simulink model "LQR"  (R2022a)
settings: Solver=VariableStepAuto  StartTime=0.0  StopTime=10.0  RelTol=1e-3
values from neighbouring files (symbols this model uses):
  dragConstants = [dx, dy, 0]    [parameters_init.m]    (also in parameters_init2.m)
  g = 9.81    [LQRCalcs.m]    (also in cf_firstOrderStateMdl.m; init_parameters.m; main.m; parameters_buildingSimulink.m)
  Gamma = [cT, cT, cT, cT ... (first row only)    [init_parameters.m]    (also in parameters_buildingSimulink.m; parameters_init.m; parameters_init2.m; parameters_init____CodeToImplementLater.m)
  GammaInv = inv(Gamma)    [init_parameters.m]    (also in parameters_buildingSimulink.m; parameters_init.m; parameters_init2.m)
  J = cat(2, [0 0 0]', J)    [LQRCalcs.m]    (also in init_parameters.m = diag([0.082, 0.0845, 0.1377]); main.m = diag([0.082, 0.0845, 0.1377]); parameters_buildingSimulink.m = diag([0.082, 0.0845, 0.1377]); parameters_init.m = Crazyflie.J)
  J_inv = inv(J)    [main.m]    (also in parameters_init.m; parameters_init2.m)
  m = 0.003    [LQRCalcs.m]    (also in cf_firstOrderStateMdl.m; init_parameters.m = 4.34; main.m = 4.34; parameters_buildingSimulink.m = 4.34)
  projectionMatrix = [1, 0, 0; 0, 1, 0]    [parameters_init.m]    (also in parameters_init2.m)
undefined symbols (not defined in the file or in its folder): Gain, sigbuilder_block
libraries: matrix_library x2, aerolibutil x2, sharedtransform x2
settings Model: Creator=Drew Lab Computer 1  LastModifiedBy=Drew Lab Computer 1

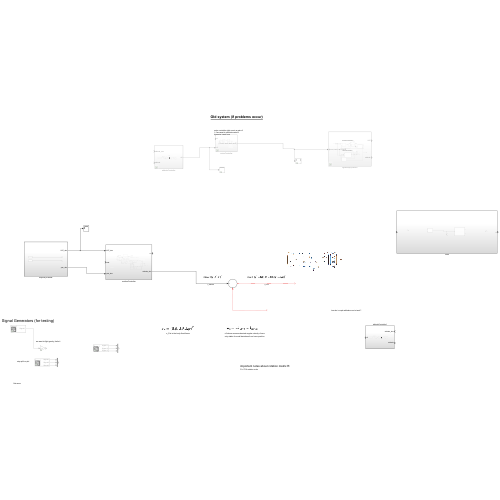
[thumbnail: Simulink's stored preview of the top-level diagram]
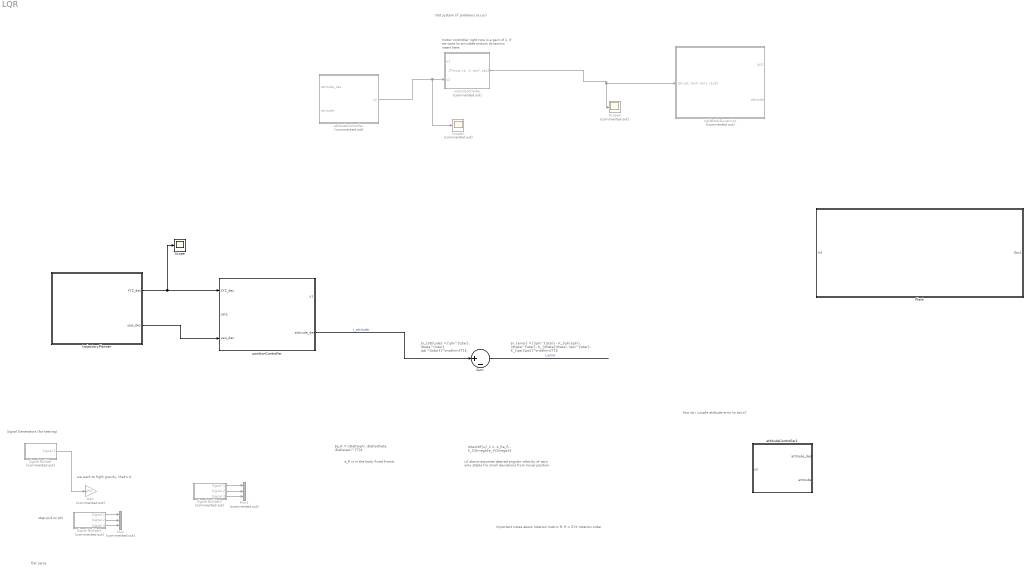
== system LQR ==
  note: $r_{attitude} = [\phi^{\star}, \theta^{\star}, \psi^{\star}]^\mathrm{T}$
  note: Old system (if problems occur)
  note: we want to fight gravity, that's it
  note: Signal Generators (for testing)
  note: flat zeros
  note: step pi/4 on phi
  note: $\textbf{u}_2 = -k_Re_R - k_{\Omega}e_{\Omega}$
  note: motor controller right now is a gain of 1, if we want to simulate motors dynamics insert here
  note: $e_R = (\Delta\phi, \Delta\theta, \Delta\psi)^{T}$
  note: $r_{error} = [(\phi^{\star} - K_{\phi}\phi), (\theta^{\star}- K_{\theta}\theta), (\psi^{\star}- K_{\psi}\psi)]^\mathrm{T}$
  note: u2 above assumes desired angular velocity of zero
      | only stable fro small deviations from hover position
  note: how do i couple attitude error to tau's?
  note: important notes about rotation matrix R:
      | R = ZYX rotation order
  note: e_R is in the body-fixed frame
  Gain : Gain  Commented=on  Gain=g*m
  Mux : Mux  Commented=on  Inputs=3
  Mux1 : Mux  Commented=on  Inputs=3
  Plant : Subsystem
  Scope : Scope
  Scope2 : Scope  Commented=on
  Scope3 : Scope  Commented=on
  Signal Builder : Subsystem  Tag=STV Subsys  Commented=on  LoadFcn=sigbuilder_block('load');  StartFcn=sigbuilder_block('start');  StopFcn=sigbuilder_block('stop');  ClipboardFcn=sigbuilder_block('clipboard');  mask(Sigbuilder block){tuvar=[0:10]}
      mask help: Simulink:masks:SigbuilderBlock_MD
      mask init:
      | if ~strcmp(get_param(bdroot(gcbh),'SimulationStatus'),'stopped') tuvar = sigbuilder_block('maskInit'); end
      settings: CopyFcn=sigbuilder_block('copy');  DeleteFcn=sigbuilder_block('delete');  ModelCloseFcn=sigbuilder_block('modelClose');  PreSaveFcn=sigbuilder_block('preSave');  PauseFcn=sigbuilder_block('pause');  ContinueFcn=sigbuilder_block('continue');  NameChangeFcn=sigbuilder_block('namechange');  OpenFcn=sigbuilder_block('open',[437.6 199.2 550.4 400 ]);  CloseFcn=sigbuilder_block('close');
      mask Display: plot(0, 0, 100, 100,[2, 2, 32, 32, 2], [68, 8, 8, 68, 68],[32, 2], [38, 38], [32, 19, 2],[53, 60, 44], [32, 17, 17, 2],[16, 16, 31, 31]);txt = getActiveGroup(gcbh);text(2, 100, txt,'verticalAlignment', 'top');
  Signal Builder1 : Subsystem  Tag=STV Subsys  Commented=on  LoadFcn=sigbuilder_block('load');  StartFcn=sigbuilder_block('start');  StopFcn=sigbuilder_block('stop');  ClipboardFcn=sigbuilder_block('clipboard');  mask(Sigbuilder block){tuvar=[0:10]}
      mask help: Simulink:masks:SigbuilderBlock_MD
      mask init:
      | if ~strcmp(get_param(bdroot(gcbh),'SimulationStatus'),'stopped') tuvar = sigbuilder_block('maskInit'); end
      settings: CopyFcn=sigbuilder_block('copy');  DeleteFcn=sigbuilder_block('delete');  ModelCloseFcn=sigbuilder_block('modelClose');  PreSaveFcn=sigbuilder_block('preSave');  PauseFcn=sigbuilder_block('pause');  ContinueFcn=sigbuilder_block('continue');  NameChangeFcn=sigbuilder_block('namechange');  OpenFcn=sigbuilder_block('open',[437.6 199.2 550.4 400 ]);  CloseFcn=sigbuilder_block('close');
      mask Display: plot(0, 0, 100, 100,[2, 2, 32, 32, 2], [68, 8, 8, 68, 68],[32, 2], [38, 38], [32, 19, 2],[53, 60, 44], [32, 17, 17, 2],[16, 16, 31, 31]);txt = getActiveGroup(gcbh);text(2, 100, txt,'verticalAlignment', 'top');
  Signal Builder2 : Subsystem  Tag=STV Subsys  Commented=on  LoadFcn=sigbuilder_block('load');  StartFcn=sigbuilder_block('start');  StopFcn=sigbuilder_block('stop');  ClipboardFcn=sigbuilder_block('clipboard');  mask(Sigbuilder block){tuvar=[0:10]}
      mask help: Simulink:masks:SigbuilderBlock_MD
      mask init:
      | if ~strcmp(get_param(bdroot(gcbh),'SimulationStatus'),'stopped') tuvar = sigbuilder_block('maskInit'); end
      settings: CopyFcn=sigbuilder_block('copy');  DeleteFcn=sigbuilder_block('delete');  ModelCloseFcn=sigbuilder_block('modelClose');  PreSaveFcn=sigbuilder_block('preSave');  PauseFcn=sigbuilder_block('pause');  ContinueFcn=sigbuilder_block('continue');  NameChangeFcn=sigbuilder_block('namechange');  OpenFcn=sigbuilder_block('open',[437.6 199.2 550.4 400 ]);  CloseFcn=sigbuilder_block('close');
      mask Display: plot(0, 0, 100, 100,[2, 2, 32, 32, 2], [68, 8, 8, 68, 68],[32, 2], [38, 38], [32, 19, 2],[53, 60, 44], [32, 17, 17, 2],[16, 16, 31, 31]);txt = getActiveGroup(gcbh);text(2, 100, txt,'verticalAlignment', 'top');
  Sum : Sum  Inputs=|+-
  attitudeController : Subsystem  Commented=on
  attitudeController1 : Subsystem
  motorController : Subsystem  Commented=on
  positionController : Subsystem
  rigidBodyDynamics : Subsystem  Commented=on
  trajectoryPlanner : Subsystem
  wires:
  Sum/1 -> ?  "r_error"
  Signal Builder/1(Signal 1) -> Gain/1
  Signal Builder2/1(Signal 1) -> Mux1/1
  Signal Builder2/3(Signal 3) -> Mux1/3
  Signal Builder2/2(Signal 2) -> Mux1/2
  trajectoryPlanner/1(XYZ_des) -> Scope/1, positionController/1(XYZ_des)
  Signal Builder1/1(Signal 1) -> Mux/1
  Signal Builder1/3(Signal 3) -> Mux/3
  positionController/2(attitude_des) -> Sum/1  "r_attitude"
  Signal Builder1/2(Signal 2) -> Mux/2
  motorController/1("[Thrust, tauX, tauY, tauZ]") -> Scope3/1, rigidBodyDynamics/1("[thrust, tauX, tauY, tauZ]")
  attitudeController/1(u2) -> Scope2/1, motorController/2(u2)
  trajectoryPlanner/2(yaw_des) -> positionController/3(yaw_des)
  ? -> Sum/2

== system LQR/Plant ==
  In1 : Inport
  Scope1 : Scope
  motorController1 : Subsystem
  rigidBodyDynamics1 : Subsystem
  Out1 : Outport
  wires:
  motorController1/1("[Thrust, tauX, tauY, tauZ]") -> Scope1/1, rigidBodyDynamics1/1("[thrust, tauX, tauY, tauZ]")

== system LQR/Signal Builder ==
  Demux : Demux  Tag=STV Demux  Outputs=1
      settings: DisplayOption=none
  FromWs : FromWorkspace  Tag=STV FromWs  VariableName=tuvar
      SigBuilderData=|
      | common.afterFinalStr = 'Extrapolate'
      | common.sampleTime = 0
      | dataSet.timeRange = [0 10]
      | dataSet.name = 'Group 1'
      | sbobj.Groups.Name = 'Group 1'
      | sbobj.Groups.Signals.Name = 'Signal 1'
      | sbobj.Groups.Signals.XData = [0 10]
      | sbobj.Groups.Signals.YData = [1 1]
  Signal 1 : Outport  Tag=STV Outport
  wires:
  Demux/1 -> Signal 1/1
  FromWs/1 -> Demux/1

== system LQR/Signal Builder1 ==
  Demux : Demux  Tag=STV Demux  Outputs=3
      settings: DisplayOption=none
  FromWs : FromWorkspace  Tag=STV FromWs  VariableName=tuvar
      SigBuilderData=|
      | common.afterFinalStr = 'Extrapolate'
      | common.sampleTime = 0
      | dataSet.timeRange = [0 10]
      | dataSet.name = 'Group 1'
      | sbobj.Groups.Name = 'Group 1'
      | sbobj.Groups.Signals(1).Name = 'Signal 1'
      | sbobj.Groups.Signals(1).XData = [0 1 1 10]
      | sbobj.Groups.Signals(1).YData = [0 0 0.1 0.1]
      | sbobj.Groups.Signals(2).Name = 'Signal 2'
      | sbobj.Groups.Signals(2).XData = [0 10]
      | sbobj.Groups.Signals(2).YData = [0 0]
      | sbobj.Groups.Signals(3).Name = 'Signal 3'
      | sbobj.Groups.Signals(3).XData = [0 10]
      | sbobj.Groups.Signals(3).YData = [0 0]
  Signal 1 : Outport  Tag=STV Outport
  Signal 2 : Outport  Tag=STV Outport  Port=2
  Signal 3 : Outport  Tag=STV Outport  Port=3
  wires:
  Demux/1 -> Signal 1/1
  FromWs/1 -> Demux/1
  Demux/2 -> Signal 2/1
  Demux/3 -> Signal 3/1

== system LQR/Signal Builder2 ==
  Demux : Demux  Tag=STV Demux  Outputs=3
      settings: DisplayOption=none
  FromWs : FromWorkspace  Tag=STV FromWs  VariableName=tuvar
      SigBuilderData=|
      | common.afterFinalStr = 'Extrapolate'
      | common.sampleTime = 0
      | dataSet.timeRange = [0 10]
      | dataSet.name = 'Group 1'
      | sbobj.Groups.Name = 'Group 1'
      | sbobj.Groups.Signals(1).Name = 'Signal 1'
      | sbobj.Groups.Signals(1).XData = [0 10]
      | sbobj.Groups.Signals(1).YData = [0 0]
      | sbobj.Groups.Signals(2).Name = 'Signal 2'
      | sbobj.Groups.Signals(2).XData = [0 10]
      | sbobj.Groups.Signals(2).YData = [0 0]
      | sbobj.Groups.Signals(3).Name = 'Signal 3'
      | sbobj.Groups.Signals(3).XData = [0 10]
      | sbobj.Groups.Signals(3).YData = [0 0]
  Signal 1 : Outport  Tag=STV Outport
  Signal 2 : Outport  Tag=STV Outport  Port=2
  Signal 3 : Outport  Tag=STV Outport  Port=3
  wires:
  Demux/1 -> Signal 1/1
  FromWs/1 -> Demux/1
  Demux/2 -> Signal 2/1
  Demux/3 -> Signal 3/1

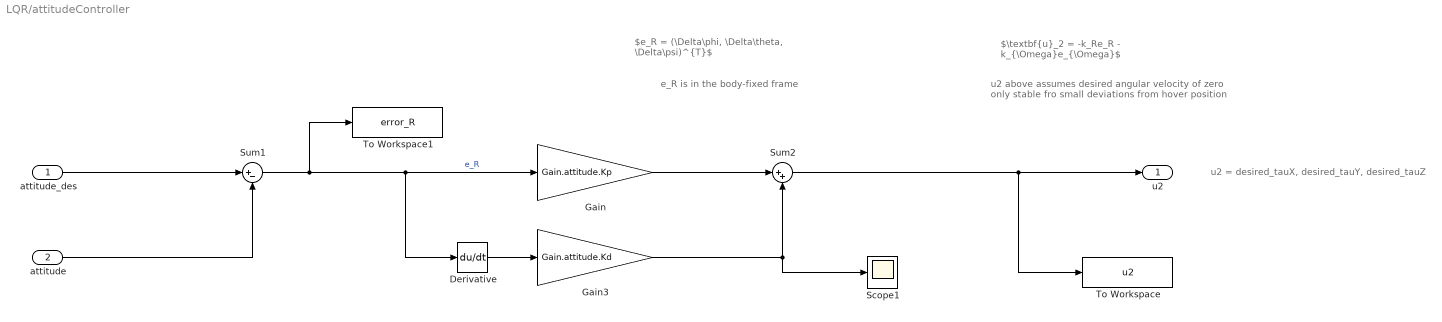
== system LQR/attitudeController ==
  note: u2 above assumes desired angular velocity of zero
      | only stable fro small deviations from hover position
  note: e_R is in the body-fixed frame
  note: $e_R = (\Delta\phi, \Delta\theta, \Delta\psi)^{T}$
  note: $\textbf{u}_2 = -k_Re_R - k_{\Omega}e_{\Omega}$
  note: u2 = desired_tauX, desired_tauY, desired_tauZ
  attitude_des : Inport
  attitude : Inport  Port=2
  Derivative : Derivative
  Gain : Gain  Gain=Gain.attitude.Kp
  Gain3 : Gain  Gain=Gain.attitude.Kd
  Scope1 : Scope
  Sum1 : Sum  Inputs=|+-
  Sum2 : Sum  Inputs=|++
  To Workspace : ToWorkspace  VariableName=u2  SaveFormat=Timeseries  SampleTime=-1
  To Workspace1 : ToWorkspace  VariableName=error_R  SaveFormat=Timeseries  SampleTime=-1
  u2 : Outport
  wires:
  attitude/1 -> Sum1/2
  Sum1/1 -> To Workspace1/1, Derivative/1, Gain/1  "e_R"
  Derivative/1 -> Gain3/1
  Gain/1 -> Sum2/1
  Gain3/1 -> Sum2/2, Scope1/1
  attitude_des/1 -> Sum1/1
  Sum2/1 -> To Workspace/1, u2/1

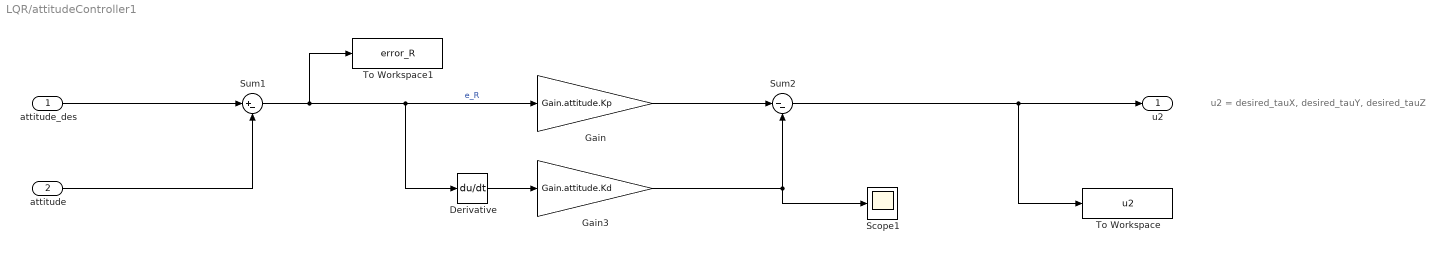
== system LQR/attitudeController1 ==
  note: u2 = desired_tauX, desired_tauY, desired_tauZ
  attitude_des : Inport
  attitude : Inport  Port=2
  Derivative : Derivative
  Gain : Gain  Gain=Gain.attitude.Kp
  Gain3 : Gain  Gain=Gain.attitude.Kd
  Scope1 : Scope
  Sum1 : Sum  Inputs=|+-
  Sum2 : Sum  Inputs=|--
  To Workspace : ToWorkspace  VariableName=u2  SaveFormat=Timeseries  SampleTime=-1
  To Workspace1 : ToWorkspace  VariableName=error_R  SaveFormat=Timeseries  SampleTime=-1
  u2 : Outport
  wires:
  attitude/1 -> Sum1/2
  Sum1/1 -> To Workspace1/1, Derivative/1, Gain/1  "e_R"
  Derivative/1 -> Gain3/1
  Gain/1 -> Sum2/1
  Gain3/1 -> Sum2/2, Scope1/1
  attitude_des/1 -> Sum1/1
  Sum2/1 -> To Workspace/1, u2/1

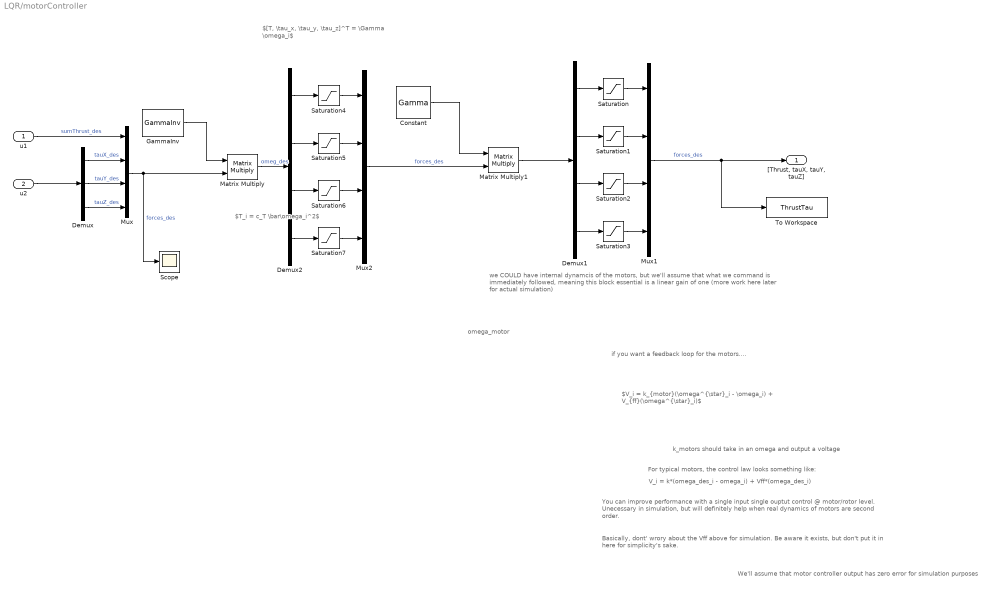
== system LQR/motorController ==
  note: $[T, \tau_x, \tau_y, \tau_z]^T = \Gamma \omega_i$
  note: if you want a feedback loop for the motors....
  note: we COULD have internal dynamcis of the motors, but we'll assume that what we command is immediately followed, meaning this block essential is a linear gain of one
      |
      | (more work here later for actual simulation)
  note: $T_i = c_T \bar\omega_i^2$
  note: omega_motor
  note: We'll assume that motor controller output has zero error for simulation purposes
  note: k_motors should take in an omega and output a voltage
  note: Basically, dont' wrory about the Vff above for simulation. Be aware it exists, but don't put it in here for simplicity's sake.
  note: You can improve performance with a single input single ouptut control @ motor/rotor level. Unecessary in simulation, but will definitely help when real dynamics of motors are second order.
  note: V_i = k*(omega_des_i - omega_i) + Vff*(omega_des_i)
  note: For typical motors, the control law looks something like:
  note: $V_i = k_{motor}(\omega^{\star}_i - \omega_i) + V_{ff}(\omega^{\star}_i)$
  u1 : Inport
  u2 : Inport  Port=2
  Constant : Constant  Value=Gamma
  Demux : Demux  Outputs=3
  Demux1 : Demux
  Demux2 : Demux
  GammaInv : Constant  Value=GammaInv
  Matrix Multiply : Product  Multiplication=Matrix(*)
  Matrix Multiply1 : Product  Multiplication=Matrix(*)
  Mux : Mux
  Mux1 : Mux
  Mux2 : Mux
  Saturation : Saturate  UpperLimit=Gain.saturation.attitude.Thrust(1)  LowerLimit=Gain.saturation.attitude.Thrust(2)
  Saturation1 : Saturate  UpperLimit=Gain.saturation.attitude.tauX(1)  LowerLimit=Gain.saturation.attitude.tauX(2)
  Saturation2 : Saturate  UpperLimit=Gain.saturation.attitude.tauY(1)  LowerLimit=Gain.saturation.attitude.tauY(2)  LinearizeAsGain=off
  Saturation3 : Saturate  UpperLimit=Gain.saturation.attitude.tauZ(1)  LowerLimit=Gain.saturation.attitude.tauZ(2)
  Saturation4 : Saturate  UpperLimit=Gain.saturation.attitude.Thrust(1)  LowerLimit=Gain.saturation.attitude.Thrust(2)
  Saturation5 : Saturate  UpperLimit=Gain.saturation.attitude.tauX(1)  LowerLimit=Gain.saturation.attitude.tauX(2)
  Saturation6 : Saturate  UpperLimit=Gain.saturation.attitude.tauY(1)  LowerLimit=Gain.saturation.attitude.tauY(2)  LinearizeAsGain=off
  Saturation7 : Saturate  UpperLimit=Gain.saturation.attitude.tauZ(1)  LowerLimit=Gain.saturation.attitude.tauZ(2)
  Scope : Scope
  To Workspace : ToWorkspace  VariableName=ThrustTau  SaveFormat=Timeseries  SampleTime=-1
  "[Thrust, tauX, tauY, tauZ]" : Outport
  wires:
  u2/1 -> Demux/1
  u1/1 -> Mux/1  "sumThrust_des"
  Demux/2 -> Mux/3  "tauY_des"
  Demux/1 -> Mux/2  "tauX_des"
  Demux/3 -> Mux/4  "tauZ_des"
  Mux/1 -> Matrix Multiply/2, Scope/1  "forces_des"
  GammaInv/1 -> Matrix Multiply/1
  Matrix Multiply/1 -> Demux2/1  "omeg_des"
  Constant/1 -> Matrix Multiply1/1
  Mux1/1 -> To Workspace/1, "[Thrust, tauX, tauY, tauZ]"/1  "forces_des"
  Demux1/1 -> Saturation/1
  Saturation/1 -> Mux1/1
  Demux1/2 -> Saturation1/1
  Demux1/3 -> Saturation2/1
  Demux1/4 -> Saturation3/1
  Saturation1/1 -> Mux1/2
  Saturation2/1 -> Mux1/3
  Saturation3/1 -> Mux1/4
  Matrix Multiply1/1 -> Demux1/1
  Demux2/2 -> Saturation5/1
  Demux2/4 -> Saturation7/1
  Saturation7/1 -> Mux2/4
  Demux2/1 -> Saturation4/1
  Demux2/3 -> Saturation6/1
  Saturation4/1 -> Mux2/1
  Saturation5/1 -> Mux2/2
  Saturation6/1 -> Mux2/3
  Mux2/1 -> Matrix Multiply1/2  "forces_des"

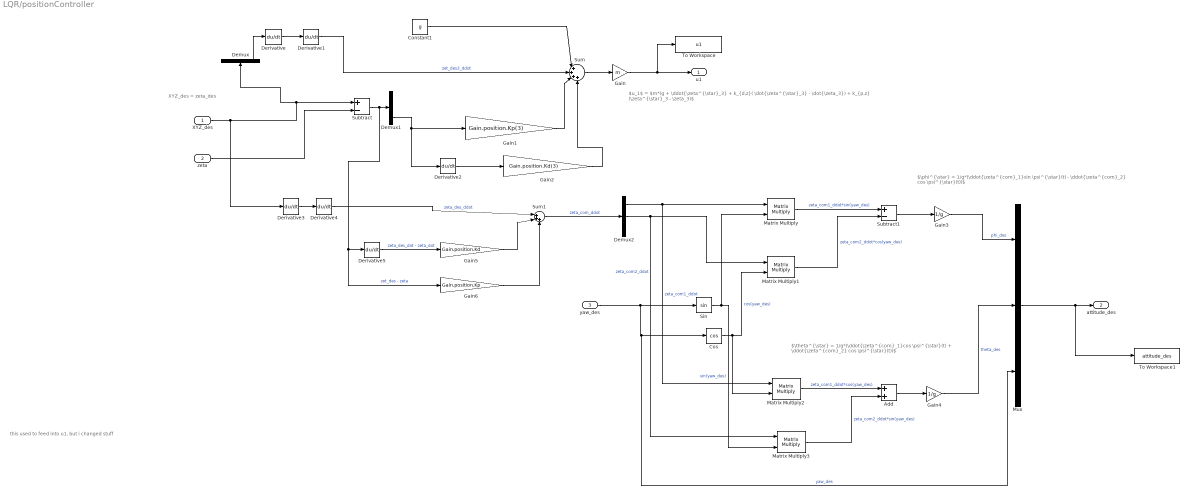
== system LQR/positionController ==
  note: $\theta^{\star} = 1/g*(\ddot{\zeta^{com}_1}cos \psi^{\star}(t) + \ddot{\zeta^{com}_2} cos \psi^{\star}(t))$
  note: $\phi^{\star} = 1/g*(\ddot{\zeta^{com}_1}sin \psi^{\star}(t) - \ddot{\zeta^{com}_2} cos \psi^{\star}(t))$
  note: XYZ_des = zeta_des
  note: $u_1$ = $m*(g + \ddot{\zeta^{\star}_3} + k_{d,z}( \dot{\zeta^{\star}_3} - \dot{\zeta_3}) + k_{p,z} (\zeta^{\star}_3 - \zeta_3)$
  note: this used to feed into u1, but i changed stuff
  XYZ_des : Inport
  zeta : Inport  Port=2
  yaw_des : Inport  Port=3
  Add : Sum
  Constant1 : Constant  Value=g
  Cos : Trigonometry  Operator=cos
  Demux : Demux  Outputs=3
  Demux1 : Demux  Outputs=3
  Demux2 : Demux  Outputs=3
  Derivative{,1..5} (6 alike) : Derivative
  Gain : Gain  Gain=m
  Gain1 : Gain  Gain=Gain.position.Kp(3)
  Gain2 : Gain  Gain=Gain.position.Kd(3)
  Gain3 : Gain  Gain=1/g
  Gain4 : Gain  Gain=1/g
  Gain5 : Gain  Gain=Gain.position.Kd
  Gain6 : Gain  Gain=Gain.position.Kp
  Matrix Multiply{,1..3} (4 alike) : Product  Multiplication=Matrix(*)
  Mux : Mux  Inputs=3
  Sin : Trigonometry
  Subtract : Sum  Inputs=+-
  Subtract1 : Sum  Inputs=+-
  Sum : Sum  Inputs=|++++
  Sum1 : Sum  Inputs=|+++
  To Workspace : ToWorkspace  VariableName=u1  SaveFormat=Timeseries  SampleTime=-1
  To Workspace1 : ToWorkspace  VariableName=attitude_des  SaveFormat=Timeseries  SampleTime=-1
  u1 : Outport
  attitude_des : Outport  Port=2
  wires:
  zeta/1 -> Subtract/2
  Sum/1 -> Gain/1
  Constant1/1 -> Sum/1
  XYZ_des/1 -> Derivative3/1, Subtract/1, Demux/1
  Demux/3 -> Derivative/1
  Derivative/1 -> Derivative1/1
  Derivative1/1 -> Sum/2  "zet_des3_ddot"
  Subtract/1 -> Gain6/1, Derivative5/1, Demux1/1  "zet_des - zeta"
  Demux1/3 -> Gain1/1, Derivative2/1
  Derivative2/1 -> Gain2/1
  Gain1/1 -> Sum/3
  Gain2/1 -> Sum/4
  Gain/1 -> To Workspace/1, u1/1
  Derivative3/1 -> Derivative4/1
  Derivative4/1 -> Sum1/1  "zeta_des_ddot"
  Derivative5/1 -> Gain5/1  "zeta_des_dot - zeta_dot"
  Gain5/1 -> Sum1/2
  Gain6/1 -> Sum1/3
  Sum1/1 -> Demux2/1  "zeta_com_ddot"
  yaw_des/1 -> Mux/3, Cos/1, Sin/1  "yaw_des"
  Demux2/1 -> Matrix Multiply2/1, Matrix Multiply/1  "zeta_com1_ddot"
  Sin/1 -> Matrix Multiply/2, Matrix Multiply3/2  "sin(yaw_des)"
  Matrix Multiply/1 -> Subtract1/1  "zeta_com1_ddot*sin(yaw_des)"
  Demux2/2 -> Matrix Multiply3/1, Matrix Multiply1/1  "zeta_com2_ddot"
  Cos/1 -> Matrix Multiply2/2, Matrix Multiply1/2  "cos(yaw_des)"
  Matrix Multiply1/1 -> Subtract1/2  "zeta_com2_ddot*cos(yaw_des)"
  Subtract1/1 -> Gain3/1
  Matrix Multiply2/1 -> Add/1  "zeta_com1_ddot*cos(yaw_des)"
  Matrix Multiply3/1 -> Add/2  "zeta_com2_ddot*sin(yaw_des)"
  Add/1 -> Gain4/1
  Gain3/1 -> Mux/1  "phi_des"
  Gain4/1 -> Mux/2  "theta_des"
  Mux/1 -> To Workspace1/1, attitude_des/1

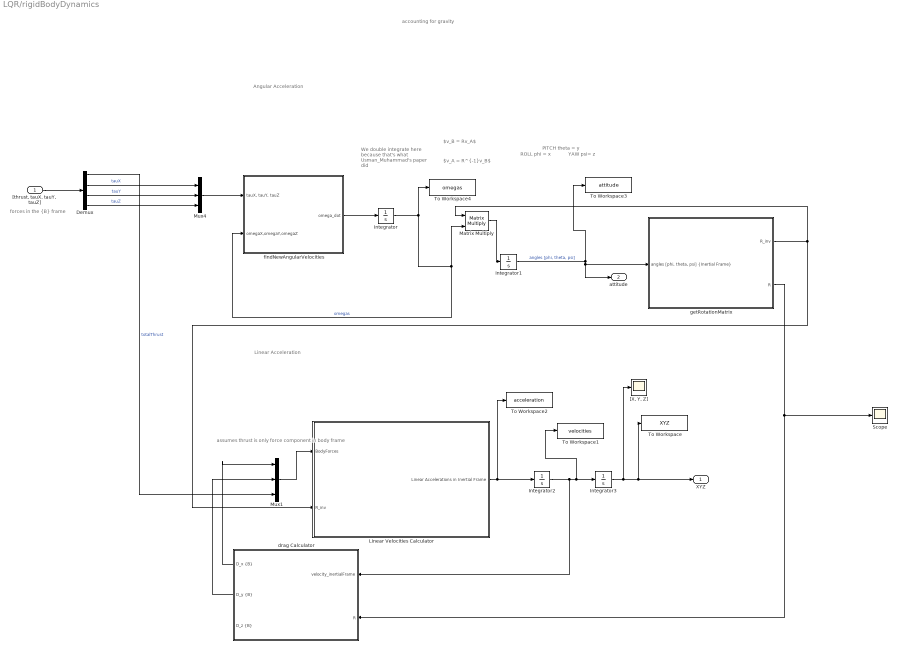
== system LQR/rigidBodyDynamics ==
  note: $v_A = R^{-1}v_B$
  note: assumes thrust is only force component in body frame
  note: We double integrate here because that's what Usman_Muhammad's paper did
  note: Angular Acceleration
  note: Linear Acceleration
  note: accounting for gravity
  note: forces in the {B} frame
  note: ROLL
      | phi = x
  note: PITCH
      | theta = y
  note: YAW
      | psi= z
  note: $v_B = Rv_A$
  "[thrust, tauX, tauY, tauZ]" : Inport
  Demux : Demux
  Integrator{,1..3} (4 alike) : Integrator
  Linear Velocities Calculator : Subsystem
  Matrix Multiply : Product  Multiplication=Matrix(*)
  Mux1 : Mux  Inputs=3
  Mux4 : Mux  Inputs=3
  Scope : Scope
  To Workspace : ToWorkspace  VariableName=XYZ  SaveFormat=Timeseries  SampleTime=-1
  To Workspace1 : ToWorkspace  VariableName=velocities  SaveFormat=Timeseries  SampleTime=-1
  To Workspace2 : ToWorkspace  VariableName=acceleration  SaveFormat=Timeseries  SampleTime=-1
  To Workspace3 : ToWorkspace  VariableName=attitude  SaveFormat=Timeseries  SampleTime=-1
  To Workspace4 : ToWorkspace  VariableName=omegas  SaveFormat=Timeseries  SampleTime=-1
  "[X, Y, Z]" : Scope
  drag Calculator : Subsystem
  findNewAngularVelocities : Subsystem
  getRotationMatrix : Subsystem
  XYZ : Outport
  attitude : Outport  Port=2
  wires:
  Demux/2 -> Mux4/1  "tauX"
  Demux/4 -> Mux4/3  "tauZ"
  Demux/3 -> Mux4/2  "tauY"
  "[thrust, tauX, tauY, tauZ]"/1 -> Demux/1
  Integrator1/1 -> attitude/1, getRotationMatrix/1("angles [phi, theta, psi] {Inertial Frame}"), To Workspace3/1  "angles [phi, theta, psi]"
  findNewAngularVelocities/1(omega_dot) -> Integrator/1
  Integrator/1 -> Matrix Multiply/2, findNewAngularVelocities/2(omegaX,omegaY,omegaZ), To Workspace4/1  "omegas"
  Mux4/1 -> findNewAngularVelocities/1("tauX, tauY, tauZ")
  Mux1/1 -> Linear Velocities Calculator/1(BodyForces)
  getRotationMatrix/1(R_inv) -> Linear Velocities Calculator/2(R_inv), Matrix Multiply/1
  Demux/1 -> Mux1/3  "totalThrust"
  Matrix Multiply/1 -> Integrator1/1
  Linear Velocities Calculator/1(Linear Accelerations in Inertial Frame) -> Integrator2/1, To Workspace2/1
  Integrator2/1 -> drag Calculator/1(velocity_inertialFrame), To Workspace1/1, Integrator3/1
  Integrator3/1 -> "[X, Y, Z]"/1, To Workspace/1, XYZ/1
  getRotationMatrix/2(R) -> Scope/1, drag Calculator/2(R)
  drag Calculator/1("D_x {B}") -> Mux1/1
  drag Calculator/2("D_y {B}") -> Mux1/2

== system LQR/trajectoryPlanner ==
  From Workspace : FromWorkspace  VariableName=zeta_des
  From Workspace1 : FromWorkspace  VariableName=yaw_des
  XYZ_des : Outport
  yaw_des : Outport  Port=2
  wires:
  From Workspace/1 -> XYZ_des/1
  From Workspace1/1 -> yaw_des/1

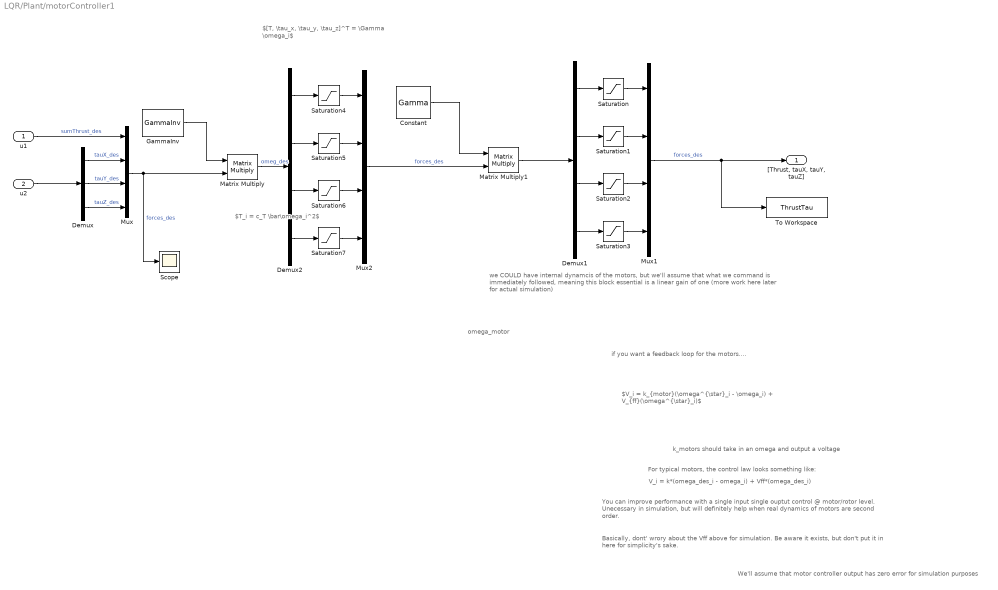
== system LQR/Plant/motorController1 ==
  note: $[T, \tau_x, \tau_y, \tau_z]^T = \Gamma \omega_i$
  note: if you want a feedback loop for the motors....
  note: we COULD have internal dynamcis of the motors, but we'll assume that what we command is immediately followed, meaning this block essential is a linear gain of one
      |
      | (more work here later for actual simulation)
  note: $T_i = c_T \bar\omega_i^2$
  note: omega_motor
  note: We'll assume that motor controller output has zero error for simulation purposes
  note: k_motors should take in an omega and output a voltage
  note: Basically, dont' wrory about the Vff above for simulation. Be aware it exists, but don't put it in here for simplicity's sake.
  note: You can improve performance with a single input single ouptut control @ motor/rotor level. Unecessary in simulation, but will definitely help when real dynamics of motors are second order.
  note: V_i = k*(omega_des_i - omega_i) + Vff*(omega_des_i)
  note: For typical motors, the control law looks something like:
  note: $V_i = k_{motor}(\omega^{\star}_i - \omega_i) + V_{ff}(\omega^{\star}_i)$
  u1 : Inport
  u2 : Inport  Port=2
  Constant : Constant  Value=Gamma
  Demux : Demux  Outputs=3
  Demux1 : Demux
  Demux2 : Demux
  GammaInv : Constant  Value=GammaInv
  Matrix Multiply : Product  Multiplication=Matrix(*)
  Matrix Multiply1 : Product  Multiplication=Matrix(*)
  Mux : Mux
  Mux1 : Mux
  Mux2 : Mux
  Saturation : Saturate  UpperLimit=Gain.saturation.attitude.Thrust(1)  LowerLimit=Gain.saturation.attitude.Thrust(2)
  Saturation1 : Saturate  UpperLimit=Gain.saturation.attitude.tauX(1)  LowerLimit=Gain.saturation.attitude.tauX(2)
  Saturation2 : Saturate  UpperLimit=Gain.saturation.attitude.tauY(1)  LowerLimit=Gain.saturation.attitude.tauY(2)  LinearizeAsGain=off
  Saturation3 : Saturate  UpperLimit=Gain.saturation.attitude.tauZ(1)  LowerLimit=Gain.saturation.attitude.tauZ(2)
  Saturation4 : Saturate  UpperLimit=Gain.saturation.attitude.Thrust(1)  LowerLimit=Gain.saturation.attitude.Thrust(2)
  Saturation5 : Saturate  UpperLimit=Gain.saturation.attitude.tauX(1)  LowerLimit=Gain.saturation.attitude.tauX(2)
  Saturation6 : Saturate  UpperLimit=Gain.saturation.attitude.tauY(1)  LowerLimit=Gain.saturation.attitude.tauY(2)  LinearizeAsGain=off
  Saturation7 : Saturate  UpperLimit=Gain.saturation.attitude.tauZ(1)  LowerLimit=Gain.saturation.attitude.tauZ(2)
  Scope : Scope
  To Workspace : ToWorkspace  VariableName=ThrustTau  SaveFormat=Timeseries  SampleTime=-1
  "[Thrust, tauX, tauY, tauZ]" : Outport
  wires:
  u2/1 -> Demux/1
  u1/1 -> Mux/1  "sumThrust_des"
  Demux/2 -> Mux/3  "tauY_des"
  Demux/1 -> Mux/2  "tauX_des"
  Demux/3 -> Mux/4  "tauZ_des"
  Mux/1 -> Matrix Multiply/2, Scope/1  "forces_des"
  GammaInv/1 -> Matrix Multiply/1
  Matrix Multiply/1 -> Demux2/1  "omeg_des"
  Constant/1 -> Matrix Multiply1/1
  Mux1/1 -> To Workspace/1, "[Thrust, tauX, tauY, tauZ]"/1  "forces_des"
  Demux1/1 -> Saturation/1
  Saturation/1 -> Mux1/1
  Demux1/2 -> Saturation1/1
  Demux1/3 -> Saturation2/1
  Demux1/4 -> Saturation3/1
  Saturation1/1 -> Mux1/2
  Saturation2/1 -> Mux1/3
  Saturation3/1 -> Mux1/4
  Matrix Multiply1/1 -> Demux1/1
  Demux2/2 -> Saturation5/1
  Demux2/4 -> Saturation7/1
  Saturation7/1 -> Mux2/4
  Demux2/1 -> Saturation4/1
  Demux2/3 -> Saturation6/1
  Saturation4/1 -> Mux2/1
  Saturation5/1 -> Mux2/2
  Saturation6/1 -> Mux2/3
  Mux2/1 -> Matrix Multiply1/2  "forces_des"

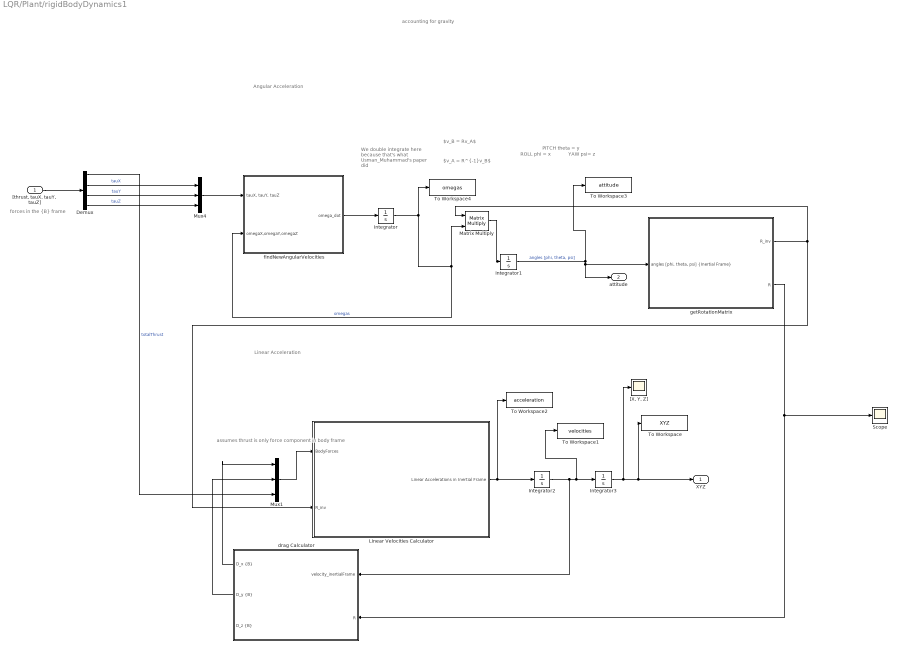
== system LQR/Plant/rigidBodyDynamics1 ==
  note: $v_A = R^{-1}v_B$
  note: assumes thrust is only force component in body frame
  note: We double integrate here because that's what Usman_Muhammad's paper did
  note: Angular Acceleration
  note: Linear Acceleration
  note: accounting for gravity
  note: forces in the {B} frame
  note: ROLL
      | phi = x
  note: PITCH
      | theta = y
  note: YAW
      | psi= z
  note: $v_B = Rv_A$
  "[thrust, tauX, tauY, tauZ]" : Inport
  Demux : Demux
  Integrator{,1..3} (4 alike) : Integrator
  Linear Velocities Calculator : Subsystem
  Matrix Multiply : Product  Multiplication=Matrix(*)
  Mux1 : Mux  Inputs=3
  Mux4 : Mux  Inputs=3
  Scope : Scope
  To Workspace : ToWorkspace  VariableName=XYZ  SaveFormat=Timeseries  SampleTime=-1
  To Workspace1 : ToWorkspace  VariableName=velocities  SaveFormat=Timeseries  SampleTime=-1
  To Workspace2 : ToWorkspace  VariableName=acceleration  SaveFormat=Timeseries  SampleTime=-1
  To Workspace3 : ToWorkspace  VariableName=attitude  SaveFormat=Timeseries  SampleTime=-1
  To Workspace4 : ToWorkspace  VariableName=omegas  SaveFormat=Timeseries  SampleTime=-1
  "[X, Y, Z]" : Scope
  drag Calculator : Subsystem
  findNewAngularVelocities : Subsystem
  getRotationMatrix : Subsystem
  XYZ : Outport
  attitude : Outport  Port=2
  wires:
  Demux/2 -> Mux4/1  "tauX"
  Demux/4 -> Mux4/3  "tauZ"
  Demux/3 -> Mux4/2  "tauY"
  "[thrust, tauX, tauY, tauZ]"/1 -> Demux/1
  Integrator1/1 -> attitude/1, getRotationMatrix/1("angles [phi, theta, psi] {Inertial Frame}"), To Workspace3/1  "angles [phi, theta, psi]"
  findNewAngularVelocities/1(omega_dot) -> Integrator/1
  Integrator/1 -> Matrix Multiply/2, findNewAngularVelocities/2(omegaX,omegaY,omegaZ), To Workspace4/1  "omegas"
  Mux4/1 -> findNewAngularVelocities/1("tauX, tauY, tauZ")
  Mux1/1 -> Linear Velocities Calculator/1(BodyForces)
  getRotationMatrix/1(R_inv) -> Linear Velocities Calculator/2(R_inv), Matrix Multiply/1
  Demux/1 -> Mux1/3  "totalThrust"
  Matrix Multiply/1 -> Integrator1/1
  Linear Velocities Calculator/1(Linear Accelerations in Inertial Frame) -> Integrator2/1, To Workspace2/1
  Integrator2/1 -> drag Calculator/1(velocity_inertialFrame), To Workspace1/1, Integrator3/1
  Integrator3/1 -> "[X, Y, Z]"/1, To Workspace/1, XYZ/1
  getRotationMatrix/2(R) -> Scope/1, drag Calculator/2(R)
  drag Calculator/1("D_x {B}") -> Mux1/1
  drag Calculator/2("D_y {B}") -> Mux1/2

== system LQR/rigidBodyDynamics/Linear Velocities Calculator ==
  note: integration for velocity calculations is outside of calculator
  note: F=ma -> F*(1/m) = a
      | We will integrate acceleration to find velocity
  note: accounting for gravity in inertial frame
  note: $\dot{v}$ = $g*\vec{a_3}$ + $1/m$ * ($RF$)$
  BodyForces : Inport
  R_inv : Inport  Port=2
  Add : Sum  Inputs=+-
  Constant : Constant  Value=g
  Demux : Demux  Outputs=3
  Gain : Gain  Gain=1/m
  Matrix Multiply : Product  Multiplication=Matrix(*)
  Mux : Mux  Inputs=3
  Linear Accelerations in Inertial Frame : Outport
  wires:
  BodyForces/1 -> Matrix Multiply/2
  R_inv/1 -> Matrix Multiply/1
  Matrix Multiply/1 -> Gain/1
  Gain/1 -> Demux/1
  Demux/3 -> Add/1
  Add/1 -> Mux/3
  Demux/2 -> Mux/2
  Demux/1 -> Mux/1
  Mux/1 -> Linear Accelerations in Inertial Frame/1
  Constant/1 -> Add/2

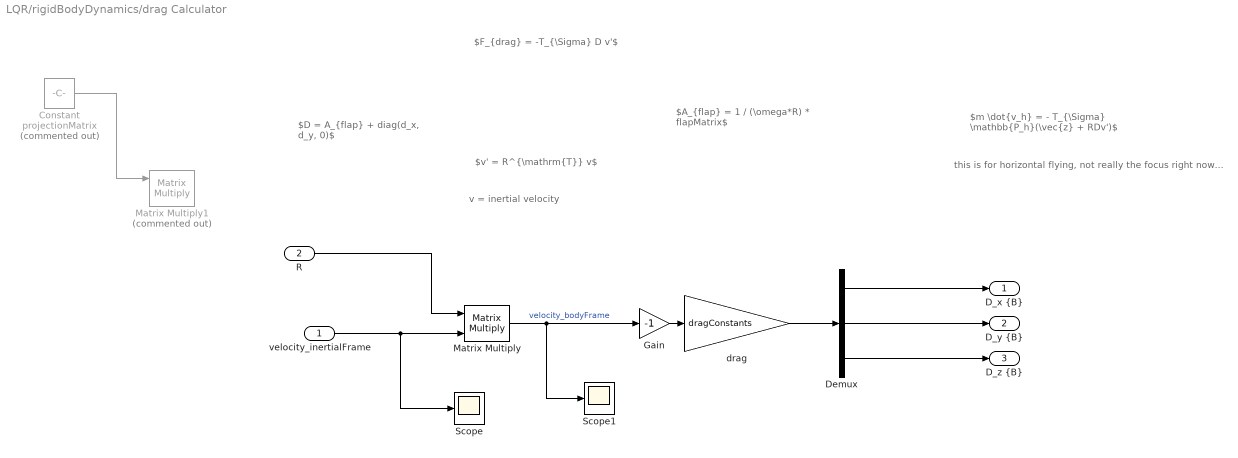
== system LQR/rigidBodyDynamics/drag Calculator ==
  note: $A_{flap} = 1 / (\omega*R) * flapMatrix$
  note: $D = A_{flap} + diag(d_x, d_y, 0)$
  note: this is for horizontal flying, not really the focus right now...
  note: $F_{drag} = -T_{\Sigma} D v'$
  note: v = inertial velocity
  note: $v' = R^{\mathrm{T}} v$
  note: $m \dot{v_h} = - T_{\Sigma} \mathbb{P_h}(\vec{z} + RDv')$
  velocity_inertialFrame : Inport
  R : Inport  Port=2
  Constant : Constant  Commented=on  Value=projectionMatrix
  Demux : Demux  Outputs=3
  Gain : Gain  Gain=-1
  Matrix Multiply : Product  Multiplication=Matrix(*)
  Matrix Multiply1 : Product  Commented=on  Multiplication=Matrix(*)
  Scope : Scope
  Scope1 : Scope
  drag : Gain  Gain=dragConstants
  "D_x {B}" : Outport
  "D_y {B}" : Outport  Port=2
  "D_z {B}" : Outport  Port=3
  wires:
  Matrix Multiply/1 -> Scope1/1, Gain/1  "velocity_bodyFrame"
  R/1 -> Matrix Multiply/1
  Demux/1 -> "D_x {B}"/1
  Demux/3 -> "D_z {B}"/1
  Gain/1 -> drag/1
  Constant/1 -> Matrix Multiply1/1
  drag/1 -> Demux/1
  Demux/2 -> "D_y {B}"/1
  velocity_inertialFrame/1 -> Scope/1, Matrix Multiply/2

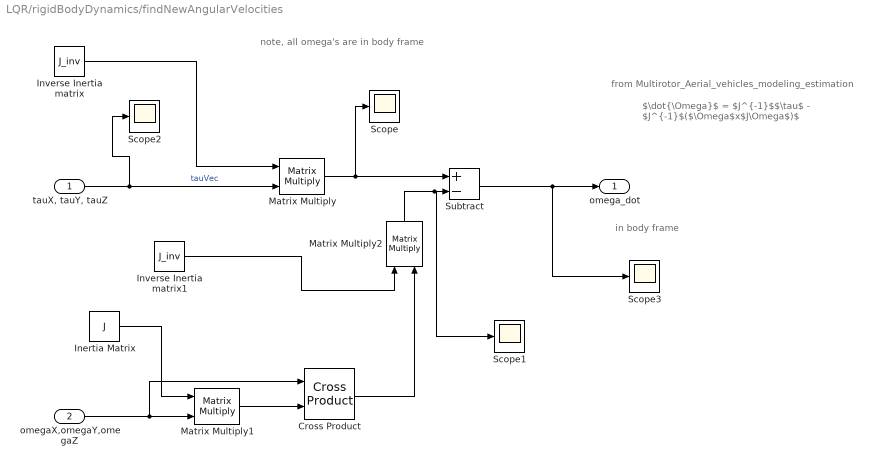
== system LQR/rigidBodyDynamics/findNewAngularVelocities ==
  note: from Multirotor_Aerial_vehicles_modeling_estimation
  note: note, all omega's are in body frame
  note: $\dot{\Omega}$ = $J^{-1}$$\tau$ - $J^{-1}$($\Omega$x$J\Omega$)$
  note: in body frame
  "tauX, tauY, tauZ" : Inport
  omegaX,omegaY,omegaZ : Inport  Port=2
  Cross Product : matrix_library/Cross Product
      settings: SourceProductBaseCode=SL
  Inertia Matrix : Constant  Value=J
  Inverse Inertia matrix : Constant  Value=J_inv
  Inverse Inertia matrix1 : Constant  Value=J_inv
  Matrix Multiply : Product  Multiplication=Matrix(*)
  Matrix Multiply1 : Product  Multiplication=Matrix(*)
  Matrix Multiply2 : Product  Multiplication=Matrix(*)
  Scope{,1..3} (4 alike) : Scope
  Subtract : Sum  Inputs=+-
  omega_dot : Outport
  wires:
  "tauX, tauY, tauZ"/1 -> Scope2/1, Matrix Multiply/2  "tauVec"
  Matrix Multiply/1 -> Scope/1, Subtract/1
  Inverse Inertia matrix/1 -> Matrix Multiply/1
  Inertia Matrix/1 -> Matrix Multiply1/1
  omegaX,omegaY,omegaZ/1 -> Cross Product/1, Matrix Multiply1/2
  Matrix Multiply1/1 -> Cross Product/2
  Inverse Inertia matrix1/1 -> Matrix Multiply2/1
  Cross Product/1 -> Matrix Multiply2/2
  Matrix Multiply2/1 -> Scope1/1, Subtract/2
  Subtract/1 -> Scope3/1, omega_dot/1

== system LQR/rigidBodyDynamics/getRotationMatrix ==
  "angles [phi, theta, psi] {Inertial Frame}" : Inport
  Invert 3x3 Matrix : aerolibutil/Invert  3x3 Matrix
  Rotation Angles to Direction Cosine Matrix : sharedtransform/Rotation Angles to Direction Cosine Matrix  rotationOrder=XYZ  aMode=aMode
      settings: SourceProductBaseCode=AE,PW,DR,MT,VE
  R_inv : Outport
  R : Outport  Port=2
  wires:
  "angles [phi, theta, psi] {Inertial Frame}"/1 -> Rotation Angles to Direction Cosine Matrix/1
  Rotation Angles to Direction Cosine Matrix/1 -> R/1, Invert 3x3 Matrix/1
  Invert 3x3 Matrix/1 -> R_inv/1

== system LQR/Plant/rigidBodyDynamics1/Linear Velocities Calculator ==
  note: integration for velocity calculations is outside of calculator
  note: F=ma -> F*(1/m) = a
      | We will integrate acceleration to find velocity
  note: accounting for gravity in inertial frame
  note: $\dot{v}$ = $g*\vec{a_3}$ + $1/m$ * ($RF$)$
  BodyForces : Inport
  R_inv : Inport  Port=2
  Add : Sum  Inputs=+-
  Constant : Constant  Value=g
  Demux : Demux  Outputs=3
  Gain : Gain  Gain=1/m
  Matrix Multiply : Product  Multiplication=Matrix(*)
  Mux : Mux  Inputs=3
  Linear Accelerations in Inertial Frame : Outport
  wires:
  BodyForces/1 -> Matrix Multiply/2
  R_inv/1 -> Matrix Multiply/1
  Matrix Multiply/1 -> Gain/1
  Gain/1 -> Demux/1
  Demux/3 -> Add/1
  Add/1 -> Mux/3
  Demux/2 -> Mux/2
  Demux/1 -> Mux/1
  Mux/1 -> Linear Accelerations in Inertial Frame/1
  Constant/1 -> Add/2

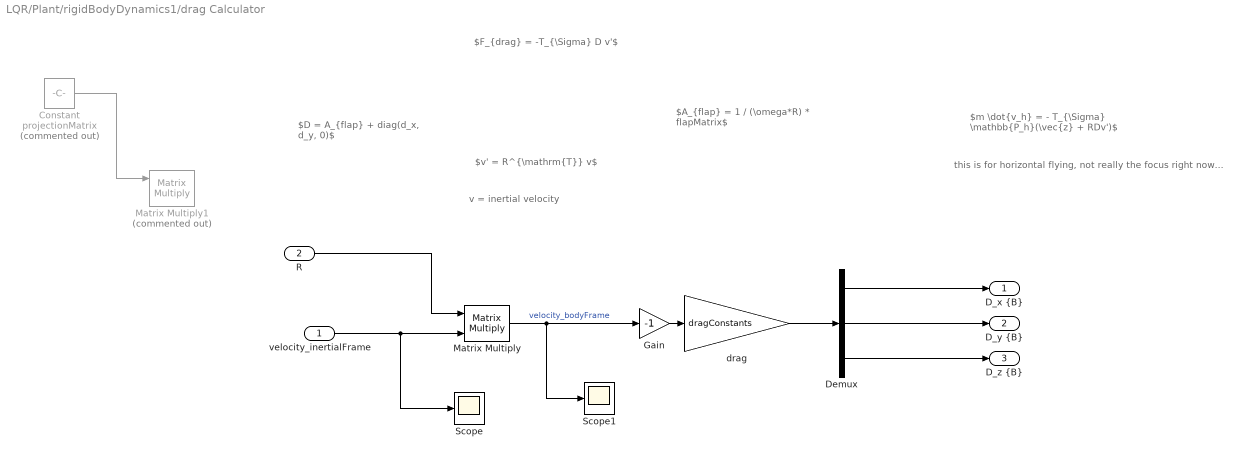
== system LQR/Plant/rigidBodyDynamics1/drag Calculator ==
  note: $A_{flap} = 1 / (\omega*R) * flapMatrix$
  note: $D = A_{flap} + diag(d_x, d_y, 0)$
  note: this is for horizontal flying, not really the focus right now...
  note: $F_{drag} = -T_{\Sigma} D v'$
  note: v = inertial velocity
  note: $v' = R^{\mathrm{T}} v$
  note: $m \dot{v_h} = - T_{\Sigma} \mathbb{P_h}(\vec{z} + RDv')$
  velocity_inertialFrame : Inport
  R : Inport  Port=2
  Constant : Constant  Commented=on  Value=projectionMatrix
  Demux : Demux  Outputs=3
  Gain : Gain  Gain=-1
  Matrix Multiply : Product  Multiplication=Matrix(*)
  Matrix Multiply1 : Product  Commented=on  Multiplication=Matrix(*)
  Scope : Scope
  Scope1 : Scope
  drag : Gain  Gain=dragConstants
  "D_x {B}" : Outport
  "D_y {B}" : Outport  Port=2
  "D_z {B}" : Outport  Port=3
  wires:
  Matrix Multiply/1 -> Scope1/1, Gain/1  "velocity_bodyFrame"
  R/1 -> Matrix Multiply/1
  Demux/1 -> "D_x {B}"/1
  Demux/3 -> "D_z {B}"/1
  Gain/1 -> drag/1
  Constant/1 -> Matrix Multiply1/1
  drag/1 -> Demux/1
  Demux/2 -> "D_y {B}"/1
  velocity_inertialFrame/1 -> Scope/1, Matrix Multiply/2

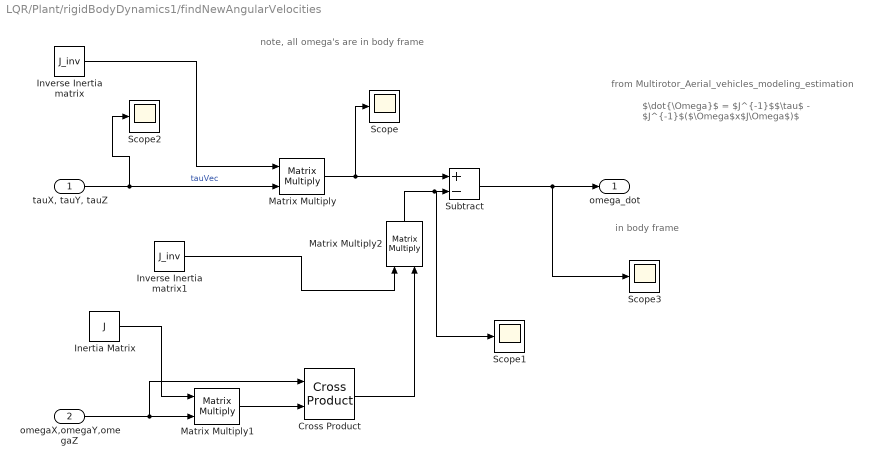
== system LQR/Plant/rigidBodyDynamics1/findNewAngularVelocities ==
  note: from Multirotor_Aerial_vehicles_modeling_estimation
  note: note, all omega's are in body frame
  note: $\dot{\Omega}$ = $J^{-1}$$\tau$ - $J^{-1}$($\Omega$x$J\Omega$)$
  note: in body frame
  "tauX, tauY, tauZ" : Inport
  omegaX,omegaY,omegaZ : Inport  Port=2
  Cross Product : matrix_library/Cross Product
      settings: SourceProductBaseCode=SL
  Inertia Matrix : Constant  Value=J
  Inverse Inertia matrix : Constant  Value=J_inv
  Inverse Inertia matrix1 : Constant  Value=J_inv
  Matrix Multiply : Product  Multiplication=Matrix(*)
  Matrix Multiply1 : Product  Multiplication=Matrix(*)
  Matrix Multiply2 : Product  Multiplication=Matrix(*)
  Scope{,1..3} (4 alike) : Scope
  Subtract : Sum  Inputs=+-
  omega_dot : Outport
  wires:
  "tauX, tauY, tauZ"/1 -> Scope2/1, Matrix Multiply/2  "tauVec"
  Matrix Multiply/1 -> Scope/1, Subtract/1
  Inverse Inertia matrix/1 -> Matrix Multiply/1
  Inertia Matrix/1 -> Matrix Multiply1/1
  omegaX,omegaY,omegaZ/1 -> Cross Product/1, Matrix Multiply1/2
  Matrix Multiply1/1 -> Cross Product/2
  Inverse Inertia matrix1/1 -> Matrix Multiply2/1
  Cross Product/1 -> Matrix Multiply2/2
  Matrix Multiply2/1 -> Scope1/1, Subtract/2
  Subtract/1 -> Scope3/1, omega_dot/1

== system LQR/Plant/rigidBodyDynamics1/getRotationMatrix ==
  "angles [phi, theta, psi] {Inertial Frame}" : Inport
  Invert 3x3 Matrix : aerolibutil/Invert  3x3 Matrix
  Rotation Angles to Direction Cosine Matrix : sharedtransform/Rotation Angles to Direction Cosine Matrix  rotationOrder=XYZ  aMode=aMode
      settings: SourceProductBaseCode=AE,PW,DR,MT,VE
  R_inv : Outport
  R : Outport  Port=2
  wires:
  "angles [phi, theta, psi] {Inertial Frame}"/1 -> Rotation Angles to Direction Cosine Matrix/1
  Rotation Angles to Direction Cosine Matrix/1 -> R/1, Invert 3x3 Matrix/1
  Invert 3x3 Matrix/1 -> R_inv/1
